simulink model "Subsystem"  (R2020a)
settings: Solver=FixedStepAuto  StartTime=0.0  StopTime=20  FixedStep=1  RelTol=1e-3
settings Model: Creator=Admin  LastModifiedBy=Admin
settings DataIOCC: SaveOutput=off  SaveTime=off

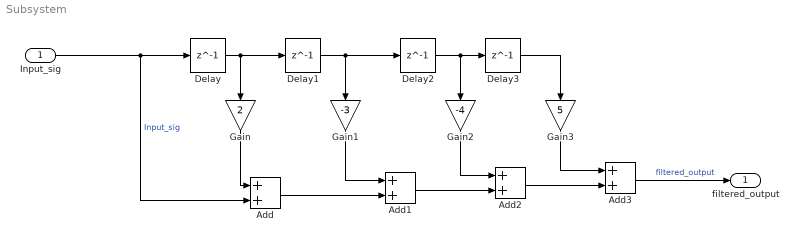
== system Subsystem ==
  Input_sig : Inport  OutDataTypeStr=double  PortDimensions=[1 1]  SampleTime=[1,0]
  Add{,1..3} (4 alike) : Sum
  Delay{,1..3} (4 alike) : Delay  DelayLength=1
  Gain : Gain  Gain=2
  Gain1 : Gain  Gain=-3
  Gain2 : Gain  Gain=-4
  Gain3 : Gain  Gain=5
  filtered_output : Outport  OutDataTypeStr=double  PortDimensions=[1 1]  SampleTime=[1,0]
  wires:
  Add1/1 -> Add2/2
  Add2/1 -> Add3/2
  Gain3/1 -> Add3/1
  Input_sig/1 -> Delay/1, Add/2  "Input_sig"
  Delay2/1 -> Delay3/1, Gain2/1
  Delay1/1 -> Delay2/1, Gain1/1
  Add/1 -> Add1/2
  Delay3/1 -> Gain3/1
  Gain/1 -> Add/1
  Delay/1 -> Delay1/1, Gain/1
  Gain1/1 -> Add1/1
  Gain2/1 -> Add2/1
  Add3/1 -> filtered_output/1  "filtered_output"
